simulink model "Copy_of_FOC_CURRENTLOOP_F103"  (R2020b)
settings: Solver=FixedStepDiscrete  StartTime=0.0  StopTime=10.0  FixedStep=TsBSP  RelTol=1e-3
values from neighbouring files (symbols this model uses):
  bandwidth = 1256.6370614359173    [Copy_of_FOC_CURRENTLOOP_F103.sldd]    (also in FOC_CURRENTLOOP_F103.sldd)
  flux = 0.0109    [Copy_of_FOC_CURRENTLOOP_F103.sldd]    (also in FOC_CURRENTLOOP_F103.sldd)
  Ls = 0.000195185    [Copy_of_FOC_CURRENTLOOP_F103.sldd]    (also in FOC_CURRENTLOOP_F103.sldd)
  Polepairs = 5.0    [Copy_of_FOC_CURRENTLOOP_F103.sldd]    (also in FOC_CURRENTLOOP_F103.sldd)
  Polepairs_MODEL = 5.0    [Copy_of_FOC_CURRENTLOOP_F103.sldd]    (also in FOC_CURRENTLOOP_F103.sldd)
  PWMHalfPeriod = 3199.0    [Copy_of_FOC_CURRENTLOOP_F103.sldd]    (also in FOC_CURRENTLOOP_F103.sldd)
  PWMHalfPeriod_MODEL = 3199.0    [Copy_of_FOC_CURRENTLOOP_F103.sldd]    (also in FOC_CURRENTLOOP_F103.sldd)
  Rs = 0.1763    [Copy_of_FOC_CURRENTLOOP_F103.sldd]    (also in FOC_CURRENTLOOP_F103.sldd)
  TsBSP = 5.0E-5    [Copy_of_FOC_CURRENTLOOP_F103.sldd]    (also in FOC_CURRENTLOOP_F103.sldd)
  TsFOC = 0.0001    [Copy_of_FOC_CURRENTLOOP_F103.sldd]    (also in FOC_CURRENTLOOP_F103.sldd)
undefined symbols (not defined in the file or in its folder): sigbuilder_block
libraries: pid_lib x2, mcbplantlib x1, simulink x1, autolibpmsmexterior x1
settings Model: DataDictionary=FOC_CURRENTLOOP_F103.sldd  Creator=beau_  LastModifiedBy=beau_
settings OptimizationCC: DefaultParameterBehavior=Inlined  EnhancedBackFolding=on  PassReuseOutputArgsAs=Individual arguments  ZeroExternalMemoryAtStartup=off  OptimizeBlockOrder=speed  DifferentSizesBufferReuse=on  OptimizationCustomize=off  EfficientTunableParamExpr=on
settings DebuggingCC: ParameterTunabilityLossMsg=error
settings HardwareCC: ProdBitPerPointer=32  ProdBitPerSizeT=32  ProdBitPerPtrDiffT=32  ProdLargestAtomicInteger=Long  ProdLargestAtomicFloat=Double  ProdWordSize=32  ProdHWDeviceType=ARM Compatible->ARM Cortex-M
settings SFSimCC: MATLABDynamicMemAlloc=off
settings RTWCC: Description=Embedded Coder  SystemTargetFile=ert.tlc  GenCodeOnly=on  TemplateMakefile=ert_default_tmf
settings CodeAppCC: ForceParamTrailComments=on  GenerateComments=off  IgnoreCustomStorageClasses=off  OperatorAnnotations=on  SimulinkDataObjDesc=on  SFDataObjDesc=on  InsertBlockDesc=on
settings ERTTargetCC: TargetLangStandard=C99 (ISO)  CodeReplacementLibrary=ARM Cortex-M  GenerateSampleERTMain=on  SupportAbsoluteTime=off  SupportNonFinite=off  SupportComplex=off  InlinedParameterPlacement=NonHierarchical  ERTCustomFileTemplate=example_file_process.tlc  IndentSize=4

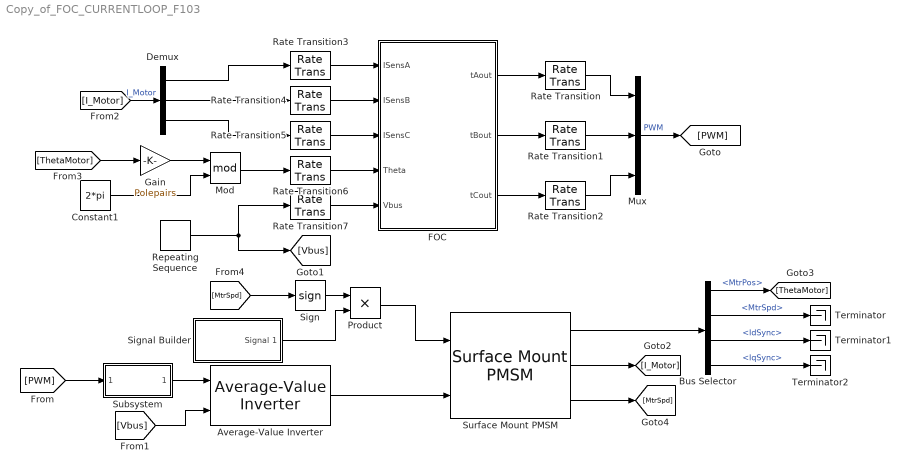
== system Copy_of_FOC_CURRENTLOOP_F103 ==
  Average-Value Inverter : mcbplantlib/Average-Value Inverter
  Bus Selector : BusSelector  OutputSignals=MtrPos,MtrSpd,IdSync,IqSync
  Constant1 : Constant  Value=2*pi
  Demux : Demux  Outputs=3
  FOC : Subsystem
  Gain : Gain  Gain=Polepairs
  Mod : Math  Operator=mod  SaturateOnIntegerOverflow=on
  Mux : Mux  Inputs=3
  Product : Product
  Rate Transition{,1..7} (8 alike) : RateTransition
  Repeating Sequence : simulink/Sources/Repeating Sequence  rep_seq_t=[0 1 2]  rep_seq_y=[20 45 20]
  Sign : Signum
  Signal Builder : Subsystem  Tag=STV Subsys  LoadFcn=sigbuilder_block('load');  StartFcn=sigbuilder_block('start');  StopFcn=sigbuilder_block('stop');  ClipboardFcn=sigbuilder_block('clipboard');  mask(Sigbuilder block){tuvar=[0:10]}
      mask help: Simulink:masks:SigbuilderBlock_MD
      mask init:
      | if ~strcmp(get_param(bdroot(gcbh),'SimulationStatus'),'stopped') tuvar = sigbuilder_block('maskInit'); end
      settings: CopyFcn=sigbuilder_block('copy');  DeleteFcn=sigbuilder_block('delete');  ModelCloseFcn=sigbuilder_block('modelClose');  PreSaveFcn=sigbuilder_block('preSave');  PauseFcn=sigbuilder_block('pause');  ContinueFcn=sigbuilder_block('continue');  NameChangeFcn=sigbuilder_block('namechange');  OpenFcn=sigbuilder_block('open',[402.75 1013.25 550.5 399.75 ]);  CloseFcn=sigbuilder_block('close');
      mask Display: plot(0, 0, 100, 100,[2, 2, 32, 32, 2], [68, 8, 8, 68, 68],[32, 2], [38, 38], [32, 19, 2],[53, 60, 44], [32, 17, 17, 2],[16, 16, 31, 31]);txt = getActiveGroup(gcbh);text(2, 100, txt,'verticalAlignment', 'top');
  Subsystem : Subsystem
  Surface Mount PMSM : autolibpmsmexterior/Surface Mount PMSM  port_config=Torque  sim_type=Discrete  Ts=TsBSP  P=Polepairs_MODEL  Rs=Rs_MODEL  Ldq_=Ls_MODEL  KConstText=Permanent flux linkage constant (lambda_pm):  lambda_pm=flux_MODEL  Ke=159.9771  Kt=1.323  mechanical=[5.8e-4, 1.59e-4, 0]  idq0=[0 0]  theta_init=0  omega_init=0  KConst=flux_MODEL  lambda_pm_calc=flux_MODEL  RefBlkName='autolibpmsmexterior/Surface Mount PMSM'  aMode=5  Ldq="[0.0017      0.0017]"
      settings: SourceProductBaseCode=PW,MT,UV,VE,VP
  Terminator : Terminator
  Terminator1 : Terminator
  Terminator2 : Terminator
  wires:
  Rate Transition3/1 -> FOC/1(ISensA)
  Rate Transition4/1 -> FOC/2(ISensB)
  Rate Transition5/1 -> FOC/3(ISensC)
  Rate Transition6/1 -> FOC/4(Theta)
  Rate Transition7/1 -> FOC/5(Vbus)
  FOC/1(tAout) -> Rate Transition/1
  FOC/2(tBout) -> Rate Transition1/1
  FOC/3(tCout) -> Rate Transition2/1
  Average-Value Inverter/1 -> Surface Mount PMSM/2
  Rate Transition1/1 -> Mux/2
  Rate Transition/1 -> Mux/1
  Rate Transition2/1 -> Mux/3
  Mux/1 -> [PWM]  "PWM"
  [PWM] -> Subsystem/1(DutyIn)
  Subsystem/1(DutyOut) -> Average-Value Inverter/1
  Repeating Sequence/1 -> Rate Transition7/1, [Vbus]
  [Vbus] -> Average-Value Inverter/2
  Surface Mount PMSM/2 -> [I_Motor]
  [I_Motor] -> Demux/1  "I_Motor"
  Demux/1 -> Rate Transition3/1
  Demux/2 -> Rate Transition4/1
  Demux/3 -> Rate Transition5/1
  Surface Mount PMSM/1 -> Bus Selector/1
  Bus Selector/1 -> [ThetaMotor]  "<MtrPos>"
  [ThetaMotor] -> Gain/1
  Gain/1 -> Mod/1
  Mod/1 -> Rate Transition6/1
  Constant1/1 -> Mod/2
  Bus Selector/2 -> Terminator/1  "<MtrSpd>"
  Bus Selector/3 -> Terminator1/1  "<IdSync>"
  Bus Selector/4 -> Terminator2/1  "<IqSync>"
  Surface Mount PMSM/3 -> [MtrSpd]
  Product/1 -> Surface Mount PMSM/1
  [MtrSpd] -> Sign/1
  Sign/1 -> Product/1
  Signal Builder/1(Signal 1) -> Product/2

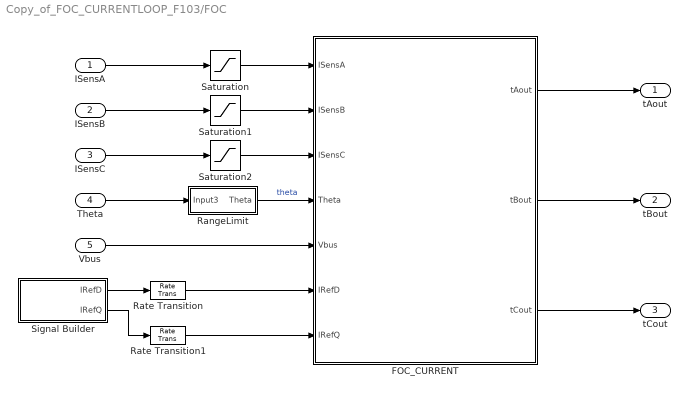
== system Copy_of_FOC_CURRENTLOOP_F103/FOC ==
  ISensA : Inport
  ISensB : Inport  Port=2
  ISensC : Inport  Port=3
  Theta : Inport  Port=4
  Vbus : Inport  Port=5
  FOC_CURRENT : Subsystem  TreatAsAtomicUnit=on  SystemSampleTime=TsFOC
  RangeLimit : Subsystem
  Rate Transition : RateTransition
  Rate Transition1 : RateTransition
  Saturation : Saturate  UpperLimit=50  LowerLimit=-50
  Saturation1 : Saturate  UpperLimit=50  LowerLimit=-50
  Saturation2 : Saturate  UpperLimit=50  LowerLimit=-50
  Signal Builder : Subsystem  Tag=STV Subsys  LoadFcn=sigbuilder_block('load');  StartFcn=sigbuilder_block('start');  StopFcn=sigbuilder_block('stop');  ClipboardFcn=sigbuilder_block('clipboard');  mask(Sigbuilder block){tuvar=[0:10]}
      mask help: Simulink:masks:SigbuilderBlock_MD
      mask init:
      | if ~strcmp(get_param(bdroot(gcbh),'SimulationStatus'),'stopped') tuvar = sigbuilder_block('maskInit'); end
      settings: CopyFcn=sigbuilder_block('copy');  DeleteFcn=sigbuilder_block('delete');  ModelCloseFcn=sigbuilder_block('modelClose');  PreSaveFcn=sigbuilder_block('preSave');  PauseFcn=sigbuilder_block('pause');  ContinueFcn=sigbuilder_block('continue');  NameChangeFcn=sigbuilder_block('namechange');  OpenFcn=sigbuilder_block('open',[413.25 918.75 550.5 358.5 ]);  CloseFcn=sigbuilder_block('close');
      mask Display: plot(0, 0, 100, 100,[2, 2, 32, 32, 2], [68, 8, 8, 68, 68],[32, 2], [38, 38], [32, 19, 2],[53, 60, 44], [32, 17, 17, 2],[16, 16, 31, 31]);txt = getActiveGroup(gcbh);text(2, 100, txt,'verticalAlignment', 'top');
  tAout : Outport
  tBout : Outport  Port=2
  tCout : Outport  Port=3
  wires:
  Vbus/1 -> FOC_CURRENT/5(Vbus)
  Saturation2/1 -> FOC_CURRENT/3(ISensC)
  Theta/1 -> RangeLimit/1(Input3)
  ISensC/1 -> Saturation2/1
  ISensB/1 -> Saturation1/1
  RangeLimit/1(Theta) -> FOC_CURRENT/4(Theta)  "theta"
  FOC_CURRENT/1(tAout) -> tAout/1
  Saturation/1 -> FOC_CURRENT/1(ISensA)
  FOC_CURRENT/2(tBout) -> tBout/1
  FOC_CURRENT/3(tCout) -> tCout/1
  Saturation1/1 -> FOC_CURRENT/2(ISensB)
  ISensA/1 -> Saturation/1
  Signal Builder/1(IRefD) -> Rate Transition/1
  Signal Builder/2(IRefQ) -> Rate Transition1/1
  Rate Transition/1 -> FOC_CURRENT/6(IRefD)
  Rate Transition1/1 -> FOC_CURRENT/7(IRefQ)

== system Copy_of_FOC_CURRENTLOOP_F103/Signal Builder ==
  Demux : Demux  Tag=STV Demux  Outputs=1
      settings: DisplayOption=none
  FromWs : FromWorkspace  Tag=STV FromWs  VariableName=tuvar
      SigBuilderData=|
      | common.afterFinalStr = 'Extrapolate'
      | common.sampleTime = 0
      | dataSet.timeRange = [0 10]
      | dataSet.name = 'Group 1'
      | sbobj.Groups.Name = 'Group 1'
      | sbobj.Groups.Signals.Name = 'Signal 1'
      | sbobj.Groups.Signals.XData = [0 0.6 0.6 1.64 1.64 2.46 2.46 4 4 5.3 5.3 6 6 7.54 8.76 10]
      | sbobj.Groups.Signals.YData = [0 0 1.5 1.5 0.1 0.1 0 0 0.62 0.62 1.5 1.5 0 0.81 0 0]
  Signal 1 : Outport  Tag=STV Outport
  wires:
  Demux/1 -> Signal 1/1
  FromWs/1 -> Demux/1

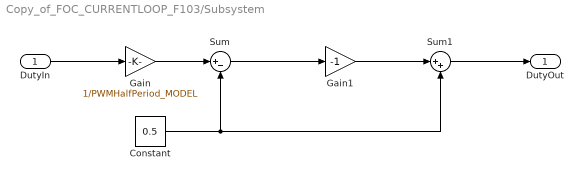
== system Copy_of_FOC_CURRENTLOOP_F103/Subsystem ==
  DutyIn : Inport
  Constant : Constant  Value=0.5
  Gain : Gain  Gain=1/PWMHalfPeriod_MODEL
  Gain1 : Gain  Gain=-1
  Sum : Sum  Inputs=|+-
  Sum1 : Sum  Inputs=|++
  DutyOut : Outport
  wires:
  DutyIn/1 -> Gain/1
  Gain/1 -> Sum/1
  Sum/1 -> Gain1/1
  Gain1/1 -> Sum1/1
  Sum1/1 -> DutyOut/1
  Constant/1 -> Sum1/2, Sum/2

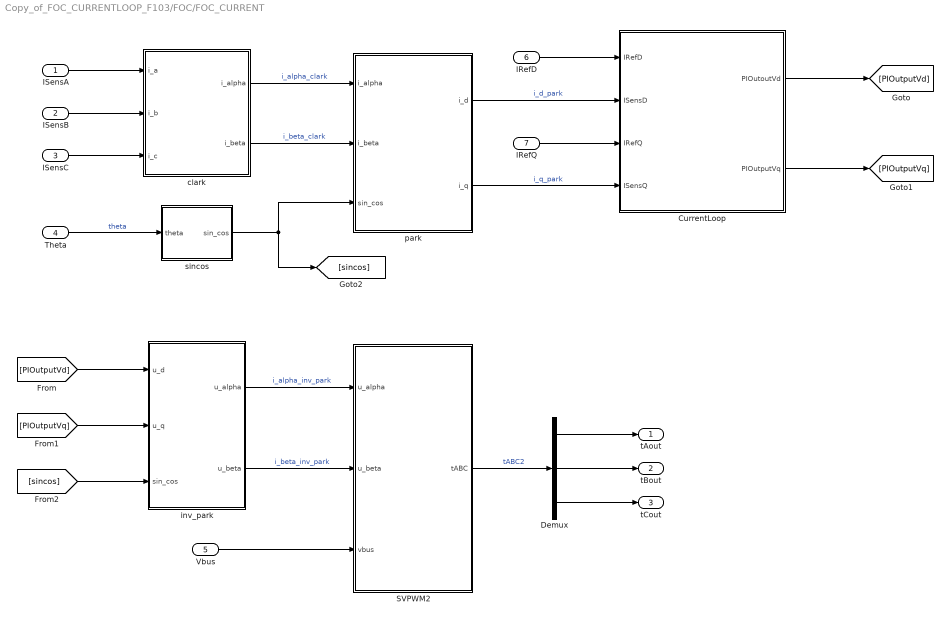
== system Copy_of_FOC_CURRENTLOOP_F103/FOC/FOC_CURRENT ==
  ISensA : Inport  OutMin=-100  OutMax=100
  ISensB : Inport  Port=2  OutMin=-100  OutMax=100
  ISensC : Inport  Port=3  OutMin=-100  OutMax=100
  Theta : Inport  Port=4  OutMin=0  OutMax=2*pi
  Vbus : Inport  Port=5  OutMin=0  OutMax=100
  IRefD : Inport  Port=6  OutMin=-50  OutMax=50
  IRefQ : Inport  Port=7  OutMin=-50  OutMax=50
  CurrentLoop : Subsystem
  Demux : Demux  Outputs=3
  SVPWM2 : Subsystem
  clark : Subsystem  TreatAsAtomicUnit=on
      mask Display:
      | port_label('input',1,'a','texmode','on');
      | port_label('input',2,'b','texmode','on');
      | port_label('input',3,'c','texmode','on');
      | 
      | port_label('output',1,'\alpha','texmode','on');
      | port_label('output',2,'\beta','texmode','on');
      | 
      | fprintf('Clark');
  inv_park : Subsystem
  park : Subsystem
  sincos : Subsystem
  tAout : Outport
  tBout : Outport  Port=2
  tCout : Outport  Port=3
  wires:
  ISensA/1 -> clark/1(i_a)
  ISensB/1 -> clark/2(i_b)
  ISensC/1 -> clark/3(i_c)
  clark/1(i_alpha) -> park/1(i_alpha)  "i_alpha_clark"
  clark/2(i_beta) -> park/2(i_beta)  "i_beta_clark"
  Theta/1 -> sincos/1(theta)  "theta"
  sincos/1(sin_cos) -> [sincos], park/3(sin_cos)
  park/1(i_d) -> CurrentLoop/2(ISensD)  "i_d_park"
  park/2(i_q) -> CurrentLoop/4(ISensQ)  "i_q_park"
  IRefD/1 -> CurrentLoop/1(IRefD)
  IRefQ/1 -> CurrentLoop/3(IRefQ)
  CurrentLoop/1(PIOutoutVd) -> [PIOutputVd]
  CurrentLoop/2(PIOutputVq) -> [PIOutputVq]
  [PIOutputVd] -> inv_park/1(u_d)
  [PIOutputVq] -> inv_park/2(u_q)
  [sincos] -> inv_park/3(sin_cos)
  inv_park/1(u_alpha) -> SVPWM2/1(u_alpha)  "i_alpha_inv_park"
  inv_park/2(u_beta) -> SVPWM2/2(u_beta)  "i_beta_inv_park"
  Vbus/1 -> SVPWM2/3(vbus)
  SVPWM2/1(tABC) -> Demux/1  "tABC2"
  Demux/1 -> tAout/1
  Demux/2 -> tBout/1
  Demux/3 -> tCout/1

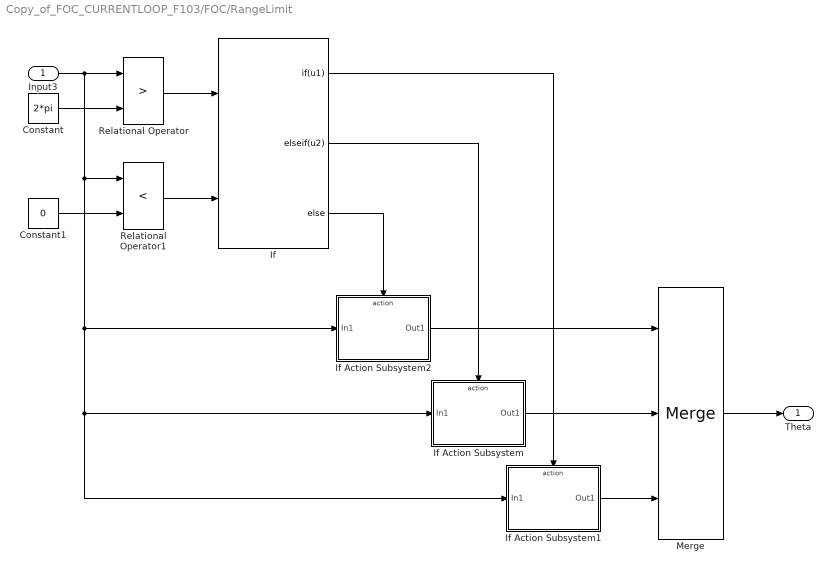
== system Copy_of_FOC_CURRENTLOOP_F103/FOC/RangeLimit ==
  Input3 : Inport
  Constant : Constant  Value=2*pi  OutDataTypeStr=double  SampleTime=-1
  Constant1 : Constant  Value=0  OutDataTypeStr=double  SampleTime=-1
  If : If  NumInputs=2  IfExpression=u1  ElseIfExpressions=u2
  If Action Subsystem : Subsystem  TreatAsAtomicUnit=on
  If Action Subsystem1 : Subsystem  TreatAsAtomicUnit=on
  If Action Subsystem2 : Subsystem  TreatAsAtomicUnit=on
  Merge : Merge  Inputs=3
  Relational Operator : RelationalOperator  Operator=>  OutDataTypeStr=boolean  RndMeth=Simplest
  Relational Operator1 : RelationalOperator  Operator=<  OutDataTypeStr=boolean  RndMeth=Simplest
  Theta : Outport
  wires:
  Relational Operator/1 -> If/1
  Constant/1 -> Relational Operator/2
  Constant1/1 -> Relational Operator1/2
  Input3/1 -> Relational Operator1/1, If Action Subsystem2/1(In1), If Action Subsystem1/1(In1), If Action Subsystem/1(In1), Relational Operator/1
  Relational Operator1/1 -> If/2
  Merge/1 -> Theta/1
  If/3 -> If Action Subsystem2/Action
  If/2 -> If Action Subsystem/Action
  If/1 -> If Action Subsystem1/Action
  If Action Subsystem2/1(Out1) -> Merge/1
  If Action Subsystem/1(Out1) -> Merge/2
  If Action Subsystem1/1(Out1) -> Merge/3

== system Copy_of_FOC_CURRENTLOOP_F103/FOC/Signal Builder ==
  Demux : Demux  Tag=STV Demux  Outputs=2
      settings: DisplayOption=none
  FromWs : FromWorkspace  Tag=STV FromWs  VariableName=tuvar
      SigBuilderData=|
      | common.afterFinalStr = 'Extrapolate'
      | common.sampleTime = 0
      | dataSet.timeRange = [0 10]
      | dataSet.name = 'Group 1'
      | sbobj.Groups.Name = 'Group 1'
      | sbobj.Groups.Signals(1).Name = 'IRefD'
      | sbobj.Groups.Signals(1).XData = [0 1.98 1.98 2.84 2.84 4 4 5 5 6 6 8 10]
      | sbobj.Groups.Signals(1).YData = [4.4 4.4 0.1 0.1 -5.1 -5.1 3.7 3.7 -0.1 -0.1 -5.5 2.9 -6]
      | sbobj.Groups.Signals(2).Name = 'IRefQ'
      | sbobj.Groups.Signals(2).XData = [0 0.72 0.72 1.74 1.74 2.28 2.28 3.28 3.28 5.18 5.18 6.62 7.62 8.8 10]
      | sbobj.Groups.Signals(2).YData = [-20 -20 20 20 0 0 9 9 -12.5 -12.5 18.5 0 15.5 -14 15]
  IRefD : Outport  Tag=STV Outport
  IRefQ : Outport  Tag=STV Outport  Port=2
  wires:
  Demux/1 -> IRefD/1
  FromWs/1 -> Demux/1
  Demux/2 -> IRefQ/1

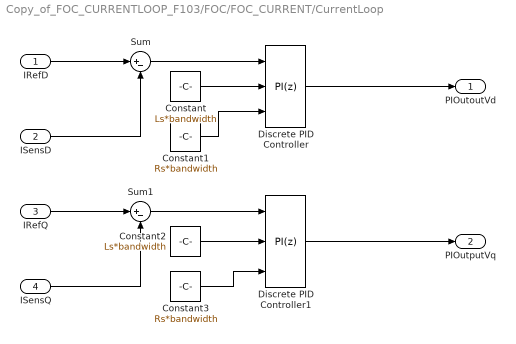
== system Copy_of_FOC_CURRENTLOOP_F103/FOC/FOC_CURRENT/CurrentLoop ==
  IRefD : Inport
  ISensD : Inport  Port=2
  IRefQ : Inport  Port=3
  ISensQ : Inport  Port=4
  Constant : Constant  Value=Ls*bandwidth  SampleTime=-1
  Constant1 : Constant  Value=Rs*bandwidth  SampleTime=-1
  Constant2 : Constant  Value=Ls*bandwidth  SampleTime=-1
  Constant3 : Constant  Value=Rs*bandwidth  SampleTime=-1
  Discrete PID Controller : pid_lib/PID Controller  Controller=PI  Form=Parallel  TimeDomain=Discrete-time  UseExternalTs=off  SampleTime=-1  IntegratorMethod=Forward Euler  FilterMethod=Forward Euler  ControllerParametersSource=external  P=1  I=1  D=0  UseFilter=on  N=100  TunerSelectOption=Transfer Function Based (PID Tuner App)  InitialConditionSource=internal  InitialConditionForIntegrator=0  InitialConditionForFilter=0  DifferentiatorICPrevScaledInput=0  ExternalReset=none  TrackingMode=off  Kt=1  LimitOutput=on  SatLimitsSource=internal  UpperSaturationLimit=10  LowerSaturationLimit=-10  LinearizeAsGain=off  AntiWindupMode=clamping  Kb=1  POutMin=[]  POutMax=[]  IOutMin=[]  IOutMax=[]  DOutMin=[]  DOutMax=[]  NOutMin=[]  NOutMax=[]  SumOutMin=[]  SumOutMax=[]  SaturationOutMin=[]  SaturationOutMax=[]  PParamMin=[]  PParamMax=[]  IParamMin=[]  IParamMax=[]  DParamMin=[]  DParamMax=[]  NParamMin=[]  NParamMax=[]  KbParamMin=[]  KbParamMax=[]  KtParamMin=[]  KtParamMax=[]  KbOutMin=[]  KbOutMax=[]  KtOutMin=[]  KtOutMax=[]  IntegratorOutMin=[]  IntegratorOutMax=[]  FilterOutMin=[]  FilterOutMax=[]  SumI1OutMin=[]  SumI1OutMax=[]  SumI2OutMin=[]  SumI2OutMax=[]  SumI3OutMin=[]  SumI3OutMax=[]  SumI4OutMin=[]  SumI4OutMax=[]  SumDOutMin=[]  SumDOutMax=[]  DifferentiatorOutMin=[]  DifferentiatorOutMax=[]  FilterDiffOutCoefMin=[]  FilterDiffOutCoefMax=[]  ReciprocalOutMin=[]  ReciprocalOutMax=[]  SumDenOutMin=[]  SumDenOutMax=[]  SumNumOutMin=[]  SumNumOutMax=[]  DivideOutMin=[]  DivideOutMax=[]  UdiffTsProdOutMin=[]  UdiffTsProdOutMax=[]  NTsProdOutMin=[]  NTsProdOutMax=[]  UintegralTsProdOutMin=[]  UintegralTsProdOutMax=[]  UngainTsProdOutMin=[]  UngainTsProdOutMax=[]  IntegratorContinuousStateAttributes=''  IntegratorStateMustResolveToSignalObject=off  IntegratorRTWStateStorageClass=Auto  FilterContinuousStateAttributes=''  FilterStateMustResolveToSignalObject=off  FilterRTWStateStorageClass=Auto  ParallelPVariant=ExternalParameters  IdealPVariant=Disabled  IVariant=ExternalParameters  DVariant=Disabled  IntegratorVariant=Discrete  SatVariant=Enabled  AWVariant=DiscClampingParallel  PCopyVariant=Disabled  TRVariant=Disabled  FdbkBlocksVariant=Forward  IdealPFdbkVariant=Disabled  SatFdbkVariant=Disabled  DerivativeFilterVariant=Disabled  NVariant=Disabled  NCopyVariant=Disabled_SignalSpec  FilterICVariant=Disabled  IntegratorICVariant=InternalICs  ExternalResetVariant=Disabled  TRSumVariant=Passthrough  SumFdbkVariant=Disabled  SumVariant=Sum_PI  TsampFilterVariant=InternalTs  TsampNgainVariant=Passthrough  TsampIntegralVariant=Passthrough  ExternalSaturationOutDataTypeStr=Inherit: Same as second input
  Discrete PID Controller1 : pid_lib/PID Controller  Controller=PI  Form=Parallel  TimeDomain=Discrete-time  UseExternalTs=off  SampleTime=-1  IntegratorMethod=Forward Euler  FilterMethod=Forward Euler  ControllerParametersSource=external  P=1  I=1  D=0  UseFilter=on  N=100  TunerSelectOption=Transfer Function Based (PID Tuner App)  InitialConditionSource=internal  InitialConditionForIntegrator=0  InitialConditionForFilter=0  DifferentiatorICPrevScaledInput=0  ExternalReset=none  TrackingMode=off  Kt=1  LimitOutput=on  SatLimitsSource=internal  UpperSaturationLimit=10  LowerSaturationLimit=-10  LinearizeAsGain=off  AntiWindupMode=clamping  Kb=1  POutMin=[]  POutMax=[]  IOutMin=[]  IOutMax=[]  DOutMin=[]  DOutMax=[]  NOutMin=[]  NOutMax=[]  SumOutMin=[]  SumOutMax=[]  SaturationOutMin=[]  SaturationOutMax=[]  PParamMin=[]  PParamMax=[]  IParamMin=[]  IParamMax=[]  DParamMin=[]  DParamMax=[]  NParamMin=[]  NParamMax=[]  KbParamMin=[]  KbParamMax=[]  KtParamMin=[]  KtParamMax=[]  KbOutMin=[]  KbOutMax=[]  KtOutMin=[]  KtOutMax=[]  IntegratorOutMin=[]  IntegratorOutMax=[]  FilterOutMin=[]  FilterOutMax=[]  SumI1OutMin=[]  SumI1OutMax=[]  SumI2OutMin=[]  SumI2OutMax=[]  SumI3OutMin=[]  SumI3OutMax=[]  SumI4OutMin=[]  SumI4OutMax=[]  SumDOutMin=[]  SumDOutMax=[]  DifferentiatorOutMin=[]  DifferentiatorOutMax=[]  FilterDiffOutCoefMin=[]  FilterDiffOutCoefMax=[]  ReciprocalOutMin=[]  ReciprocalOutMax=[]  SumDenOutMin=[]  SumDenOutMax=[]  SumNumOutMin=[]  SumNumOutMax=[]  DivideOutMin=[]  DivideOutMax=[]  UdiffTsProdOutMin=[]  UdiffTsProdOutMax=[]  NTsProdOutMin=[]  NTsProdOutMax=[]  UintegralTsProdOutMin=[]  UintegralTsProdOutMax=[]  UngainTsProdOutMin=[]  UngainTsProdOutMax=[]  IntegratorContinuousStateAttributes=''  IntegratorStateMustResolveToSignalObject=off  IntegratorRTWStateStorageClass=Auto  FilterContinuousStateAttributes=''  FilterStateMustResolveToSignalObject=off  FilterRTWStateStorageClass=Auto  ParallelPVariant=ExternalParameters  IdealPVariant=Disabled  IVariant=ExternalParameters  DVariant=Disabled  IntegratorVariant=Discrete  SatVariant=Enabled  AWVariant=DiscClampingParallel  PCopyVariant=Disabled  TRVariant=Disabled  FdbkBlocksVariant=Forward  IdealPFdbkVariant=Disabled  SatFdbkVariant=Disabled  DerivativeFilterVariant=Disabled  NVariant=Disabled  NCopyVariant=Disabled_SignalSpec  FilterICVariant=Disabled  IntegratorICVariant=InternalICs  ExternalResetVariant=Disabled  TRSumVariant=Passthrough  SumFdbkVariant=Disabled  SumVariant=Sum_PI  TsampFilterVariant=InternalTs  TsampNgainVariant=Passthrough  TsampIntegralVariant=Passthrough  ExternalSaturationOutDataTypeStr=Inherit: Same as second input
  Sum : Sum  Inputs=|+-
  Sum1 : Sum  Inputs=|+-
  PIOutoutVd : Outport
  PIOutputVq : Outport  Port=2
  wires:
  IRefD/1 -> Sum/1
  ISensD/1 -> Sum/2
  IRefQ/1 -> Sum1/1
  ISensQ/1 -> Sum1/2
  Sum/1 -> Discrete PID Controller/1
  Sum1/1 -> Discrete PID Controller1/1
  Constant/1 -> Discrete PID Controller/2
  Constant1/1 -> Discrete PID Controller/3
  Constant2/1 -> Discrete PID Controller1/2
  Constant3/1 -> Discrete PID Controller1/3
  Discrete PID Controller/1 -> PIOutoutVd/1
  Discrete PID Controller1/1 -> PIOutputVq/1

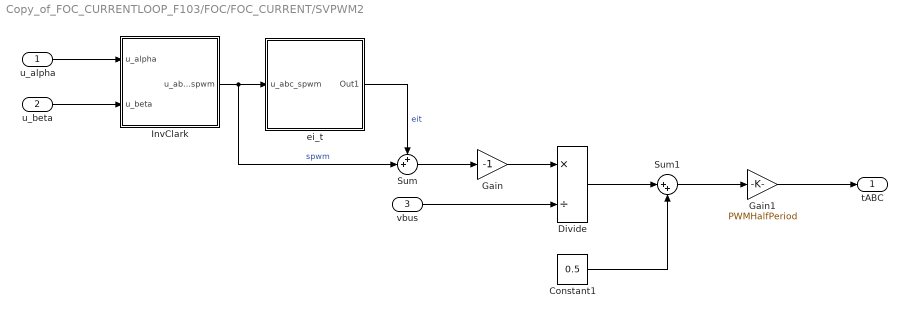
== system Copy_of_FOC_CURRENTLOOP_F103/FOC/FOC_CURRENT/SVPWM2 ==
  u_alpha : Inport
  u_beta : Inport  Port=2
  vbus : Inport  Port=3
  Constant1 : Constant  Value=0.5
  Divide : Product  Inputs=*/
  Gain : Gain  Gain=-1
  Gain1 : Gain  Gain=PWMHalfPeriod
  InvClark : Subsystem
  Sum : Sum  Inputs=++|
  Sum1 : Sum  Inputs=|++
  ei_t : Subsystem
  tABC : Outport
  wires:
  u_alpha/1 -> InvClark/1(u_alpha)
  u_beta/1 -> InvClark/2(u_beta)
  ei_t/1(Out1) -> Sum/1  "eit"
  InvClark/1(u_abc_spwm) -> Sum/2, ei_t/1(u_abc_spwm)  "spwm"
  Sum/1 -> Gain/1
  Gain/1 -> Divide/1
  vbus/1 -> Divide/2
  Divide/1 -> Sum1/1
  Constant1/1 -> Sum1/2
  Sum1/1 -> Gain1/1
  Gain1/1 -> tABC/1

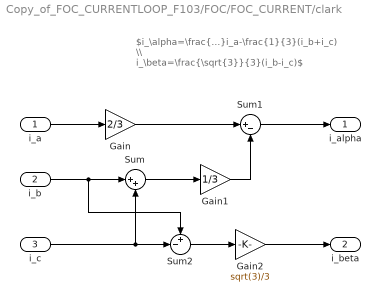
== system Copy_of_FOC_CURRENTLOOP_F103/FOC/FOC_CURRENT/clark ==
  note: $i_\alpha=\frac{2}{3}i_a-\frac{1}{3}(i_b+i_c) \\ i_\beta=\frac{\sqrt{3}}{3}(i_b-i_c)$
  i_a : Inport
  i_b : Inport  Port=2
  i_c : Inport  Port=3
  Gain : Gain  Gain=2/3
  Gain1 : Gain  Gain=1/3
  Gain2 : Gain  Gain=sqrt(3)/3
  Sum : Sum  Inputs=|++
  Sum1 : Sum  Inputs=|+-
  Sum2 : Sum  Inputs=+-|
  i_alpha : Outport
  i_beta : Outport  Port=2
  wires:
  i_b/1 -> Sum2/1, Sum/1
  Sum/1 -> Gain1/1
  i_c/1 -> Sum2/2, Sum/2
  i_a/1 -> Gain/1
  Gain/1 -> Sum1/1
  Gain1/1 -> Sum1/2
  Sum1/1 -> i_alpha/1
  Sum2/1 -> Gain2/1
  Gain2/1 -> i_beta/1

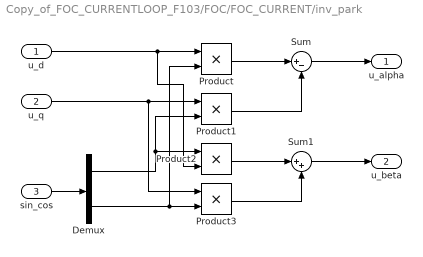
== system Copy_of_FOC_CURRENTLOOP_F103/FOC/FOC_CURRENT/inv_park ==
  u_d : Inport
  u_q : Inport  Port=2
  sin_cos : Inport  Port=3
  Demux : Demux  Outputs=2
  Product{,1..3} (4 alike) : Product
  Sum : Sum  Inputs=|+-
  Sum1 : Sum  Inputs=|++
  u_alpha : Outport
  u_beta : Outport  Port=2
  wires:
  u_d/1 -> Product2/2, Product/1
  sin_cos/1 -> Demux/1
  Demux/2 -> Product/2, Product3/2
  u_q/1 -> Product3/1, Product1/1
  Demux/1 -> Product1/2, Product2/1
  Product/1 -> Sum/1
  Product1/1 -> Sum/2
  Sum/1 -> u_alpha/1
  Product2/1 -> Sum1/1
  Product3/1 -> Sum1/2
  Sum1/1 -> u_beta/1

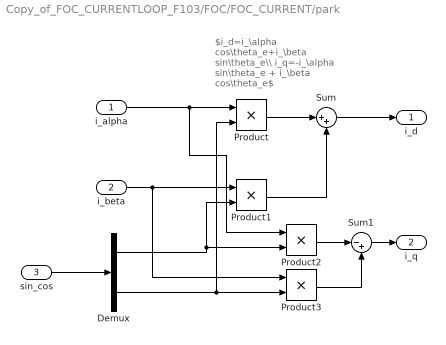
== system Copy_of_FOC_CURRENTLOOP_F103/FOC/FOC_CURRENT/park ==
  note: $i_d=i_\alpha cos\theta_e+i_\beta sin\theta_e\\ i_q=-i_\alpha sin\theta_e + i_\beta cos\theta_e$
  i_alpha : Inport
  i_beta : Inport  Port=2
  sin_cos : Inport  Port=3
  Demux : Demux  Outputs=2
  Product{,1..3} (4 alike) : Product
  Sum : Sum  Inputs=|++
  Sum1 : Sum  Inputs=|-+
  i_d : Outport
  i_q : Outport  Port=2
  wires:
  sin_cos/1 -> Demux/1
  i_alpha/1 -> Product2/1, Product/1
  Demux/2 -> Product/2, Product3/2
  Demux/1 -> Product1/2, Product2/2
  Product/1 -> Sum/1
  Product1/1 -> Sum/2
  Sum/1 -> i_d/1
  i_beta/1 -> Product3/1, Product1/1
  Product2/1 -> Sum1/1
  Product3/1 -> Sum1/2
  Sum1/1 -> i_q/1

== system Copy_of_FOC_CURRENTLOOP_F103/FOC/FOC_CURRENT/sincos ==
  theta : Inport
  Mux : Mux  Inputs=2
  SinCos : Trigonometry  Operator=sincos
  sin_cos : Outport
  wires:
  theta/1 -> SinCos/1
  SinCos/2 -> Mux/2
  SinCos/1 -> Mux/1
  Mux/1 -> sin_cos/1

== system Copy_of_FOC_CURRENTLOOP_F103/FOC/RangeLimit/If Action Subsystem ==
  In1 : Inport
  Action Port : ActionPort  ActionPortLabel=elseif(u2)
  Constant : Constant  Value=2*pi  OutDataTypeStr=double  SampleTime=-1
  Sum : Sum  Inputs=|++
  Out1 : Outport
  wires:
  In1/1 -> Sum/1
  Constant/1 -> Sum/2
  Sum/1 -> Out1/1

== system Copy_of_FOC_CURRENTLOOP_F103/FOC/RangeLimit/If Action Subsystem1 ==
  In1 : Inport
  Action Port : ActionPort  ActionPortLabel=if(u1)
  Constant : Constant  Value=2*pi  OutDataTypeStr=double  SampleTime=-1
  Sum : Sum  Inputs=|+-
  Out1 : Outport
  wires:
  In1/1 -> Sum/1
  Constant/1 -> Sum/2
  Sum/1 -> Out1/1

== system Copy_of_FOC_CURRENTLOOP_F103/FOC/RangeLimit/If Action Subsystem2 ==
  In1 : Inport
  Action Port : ActionPort  ActionPortLabel=else
  Out1 : Outport
  wires:
  In1/1 -> Out1/1

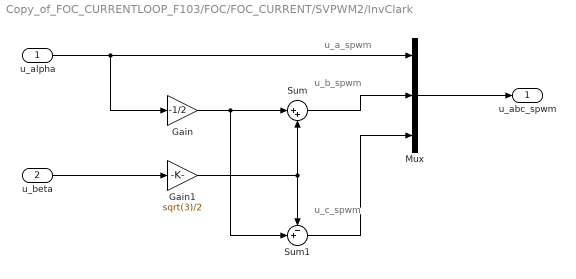
== system Copy_of_FOC_CURRENTLOOP_F103/FOC/FOC_CURRENT/SVPWM2/InvClark ==
  note: u_a_spwm
  note: u_b_spwm
  note: u_c_spwm
  u_alpha : Inport
  u_beta : Inport  Port=2
  Gain : Gain  Gain=-1/2
  Gain1 : Gain  Gain=sqrt(3)/2
  Mux : Mux  Inputs=3
  Sum : Sum  Inputs=|++
  Sum1 : Sum  Inputs=-+|
  u_abc_spwm : Outport
  wires:
  Gain/1 -> Sum1/2, Sum/1
  u_beta/1 -> Gain1/1
  Gain1/1 -> Sum1/1, Sum/2
  u_alpha/1 -> Mux/1, Gain/1
  Sum/1 -> Mux/2
  Sum1/1 -> Mux/3
  Mux/1 -> u_abc_spwm/1

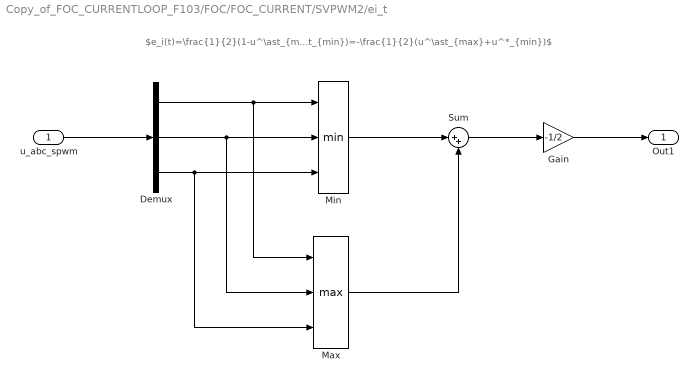
== system Copy_of_FOC_CURRENTLOOP_F103/FOC/FOC_CURRENT/SVPWM2/ei_t ==
  note: $e_i(t)=\frac{1}{2}(1-u^\ast_{max})+\frac{1}{2}(-1-u^\ast_{min})=-\frac{1}{2}(u^\ast_{max}+u^*_{min})$
  u_abc_spwm : Inport
  Demux : Demux  Outputs=3
  Gain : Gain  Gain=-1/2
  Max : MinMax  Function=max  Inputs=3
  Min : MinMax  Inputs=3
  Sum : Sum  Inputs=|++
  Out1 : Outport
  wires:
  u_abc_spwm/1 -> Demux/1
  Demux/1 -> Max/1, Min/1
  Demux/2 -> Max/2, Min/2
  Demux/3 -> Max/3, Min/3
  Min/1 -> Sum/1
  Max/1 -> Sum/2
  Sum/1 -> Gain/1
  Gain/1 -> Out1/1
